simulink model "cal_sim"  (R2016a)
settings: Solver=FixedStepAuto  StartTime=0.0  StopTime=5  FixedStep=0.01  RelTol=1e-3
undefined symbols (not defined in the file): EEP
libraries: Module_wrapper x1
settings Model: Creator=PLOCH37  LastModifiedBy=PLOCH37
settings DataIOCC: SaveOutput=off  SignalLogging=off  DSMLogging=off  SaveTime=off

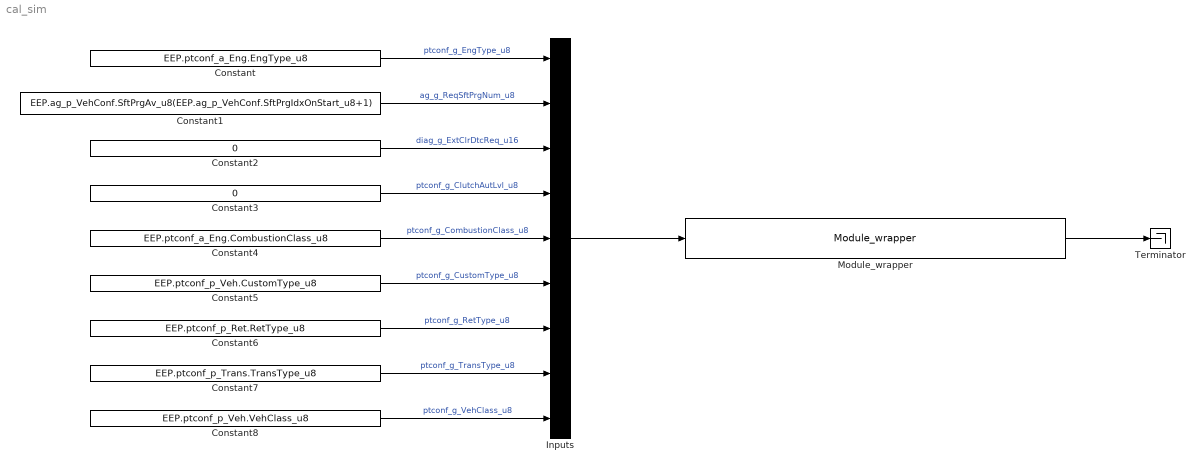
== system cal_sim ==
  Constant : Constant  Value=EEP.ptconf_a_Eng.EngType_u8
  Constant1 : Constant  Value=EEP.ag_p_VehConf.SftPrgAv_u8(EEP.ag_p_VehConf.SftPrgIdxOnStart_u8+1)
  Constant2 : Constant  Value=0
  Constant3 : Constant  Value=0
  Constant4 : Constant  Value=EEP.ptconf_a_Eng.CombustionClass_u8
  Constant5 : Constant  Value=EEP.ptconf_p_Veh.CustomType_u8
  Constant6 : Constant  Value=EEP.ptconf_p_Ret.RetType_u8
  Constant7 : Constant  Value=EEP.ptconf_p_Trans.TransType_u8
  Constant8 : Constant  Value=EEP.ptconf_p_Veh.VehClass_u8
  Inputs : BusCreator  Inputs=9
  Module_wrapper : Module_wrapper/Module_wrapper  SystemSampleTime=-1
  Terminator : Terminator
  wires:
  Constant/1 -> Inputs/1  "ptconf_g_EngType_u8"
  Constant1/1 -> Inputs/2  "ag_g_ReqSftPrgNum_u8"
  Constant2/1 -> Inputs/3  "diag_g_ExtClrDtcReq_u16"
  Constant3/1 -> Inputs/4  "ptconf_g_ClutchAutLvl_u8"
  Constant4/1 -> Inputs/5  "ptconf_g_CombustionClass_u8"
  Constant5/1 -> Inputs/6  "ptconf_g_CustomType_u8"
  Constant6/1 -> Inputs/7  "ptconf_g_RetType_u8"
  Constant7/1 -> Inputs/8  "ptconf_g_TransType_u8"
  Constant8/1 -> Inputs/9  "ptconf_g_VehClass_u8"
  Inputs/1 -> Module_wrapper/1
  Module_wrapper/1 -> Terminator/1
